simulink subsystem "Sensor_Array"  (R2022b)
settings: Solver=VariableStepAuto  StartTime=0.0  StopTime=10.0  RelTol=1e-3
model mask{input1=1, input2=2, input3=3, input4=5}
  mask prompts: input1 "Position Sensor Input:"; input2 "Velocity Sensor Input:"; input3 "Current Sensor Input:"; input4 "Voltage Sensor Input:"
settings Model: Creator=gotta  LastModifiedBy=gotta

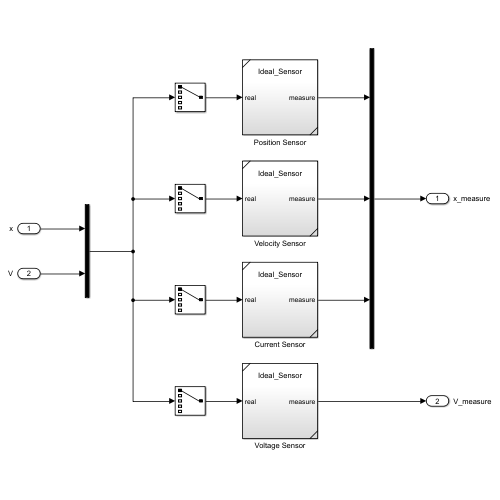
[thumbnail: Simulink's stored preview of the top-level diagram]
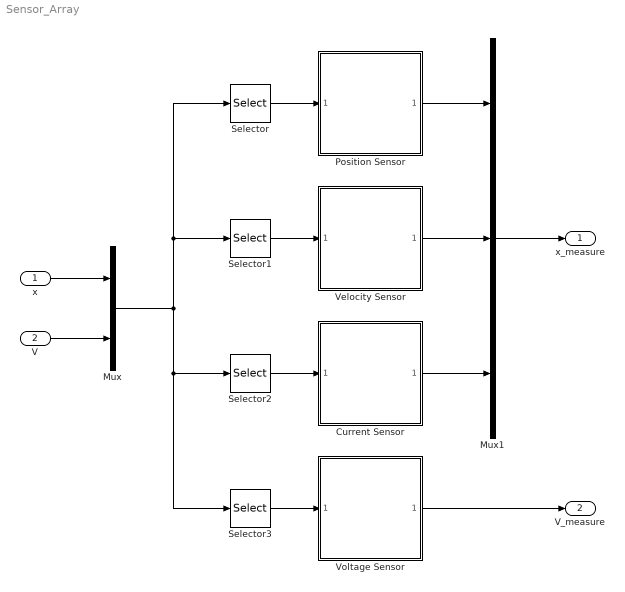
== system Sensor_Array ==
  x : Inport
  V : Inport  Port=2
  Current Sensor : Subsystem  ReferencedSubsystem=Ideal_Sensor
  Mux : Mux  Inputs=2
  Mux1 : Mux  Inputs=3
  Position Sensor : Subsystem  ReferencedSubsystem=AS5600_Sensor  sensor_model=AS5600  wrapping=off  offset=0
  Selector : Selector  InputPortWidth=4  IndexOptions=Index vector (dialog)  Indices=input1  OutputSizes=1
  Selector1 : Selector  InputPortWidth=4  IndexOptions=Index vector (dialog)  Indices=input2  OutputSizes=1
  Selector2 : Selector  InputPortWidth=4  IndexOptions=Index vector (dialog)  Indices=input3  OutputSizes=1
  Selector3 : Selector  InputPortWidth=4  IndexOptions=Index vector (dialog)  Indices=input4  OutputSizes=1
  Velocity Sensor : Subsystem  ReferencedSubsystem=Real_Derivative
  Voltage Sensor : Subsystem  ReferencedSubsystem=Ideal_Sensor
  x_measure : Outport
  V_measure : Outport  Port=2
  wires:
  x/1 -> Mux/1
  V/1 -> Mux/2
  Selector3/1 -> Voltage Sensor/1
  Selector2/1 -> Current Sensor/1
  Selector1/1 -> Velocity Sensor/1
  Selector/1 -> Position Sensor/1
  Mux/1 -> Selector/1, Selector1/1, Selector3/1, Selector2/1
  Position Sensor/1 -> Mux1/1
  Velocity Sensor/1 -> Mux1/2
  Current Sensor/1 -> Mux1/3
  Mux1/1 -> x_measure/1
  Voltage Sensor/1 -> V_measure/1
